simulink model "OneActuatorRWD"  (R2026b)
settings: Solver=VariableStepAuto
settings Model: Creator=The MathWorks, Inc.  LastModifiedBy=The MathWorks, Inc.

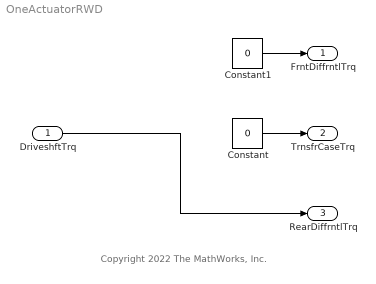
== system OneActuatorRWD ==
  note: Copyright 2022 The MathWorks, Inc.
  DriveshftTrq : Inport
  Constant : Constant  Value=0  SampleTime=-1
  Constant1 : Constant  Value=0  SampleTime=-1
  FrntDiffrntlTrq : Outport
  TrnsfrCaseTrq : Outport  Port=2
  RearDiffrntlTrq : Outport  Port=3
  wires:
  Constant/1 -> TrnsfrCaseTrq/1
  DriveshftTrq/1 -> RearDiffrntlTrq/1
  Constant1/1 -> FrntDiffrntlTrq/1
